simulink model "Labo4_students"  (R2021a)
settings: Solver=VariableStepAuto  StartTime=0.0  StopTime=30.0  RelTol=1e-3
settings Model: Creator=fwielant  LastModifiedBy=sambon
settings SolverCC: AlgebraicLoopSolver=TrustRegion
settings DataIOCC: ReturnWorkspaceOutputs=off
settings DebuggingCC: SFMachineParentedDataDiag=warning  ArithmeticOperatorsInVariantConditions=warning
settings SFSimCC: SimUseLocalCustomCode=off  CustomCodeUndefinedFunction=UseInterfaceOnly
settings RTWCC: RTWUseLocalCustomCode=off  Toolchain=MinGW64 | gmake (64-bit Windows)

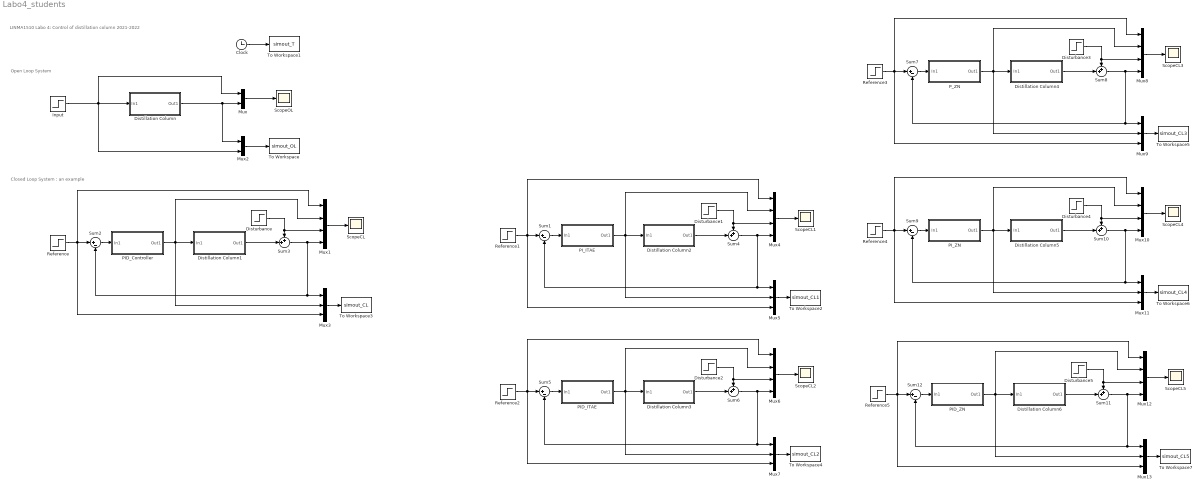
== system Labo4_students ==
  note: Open Loop System
  note: LINMA1510 Labo 4: Control of distillation column 2021-2022
  note: Closed Loop System : an example
  " PID_ITAE" : Subsystem
  Clock : Clock
  Distillation Column : Subsystem
  Distillation Column1 : Subsystem
  Distillation Column2 : Subsystem
  Distillation Column3 : Subsystem
  Distillation Column4 : Subsystem
  Distillation Column5 : Subsystem
  Distillation Column6 : Subsystem
  Disturbance{,1..5} (6 alike) : Step  Time=15  After=0.5  SampleTime=0
  Input : Step  Time=0  SampleTime=0
  Mux : Mux  Inputs=2
  Mux{1,4,6,8,10,12} (6 alike) : Mux
  Mux{3,5,7,9,11,13} (6 alike) : Mux  Inputs=3
  Mux2 : Mux  Inputs=2
  PID_Controller : Subsystem
  PID_ZN : Subsystem
  PI_ITAE : Subsystem
  PI_ZN : Subsystem
  P_ZN : Subsystem
  Reference{,1..5} (6 alike) : Step  SampleTime=0
  ScopeCL{,1..5} (6 alike) : Scope
  ScopeOL : Scope
  Sum{1..2,5,7,9,12} (6 alike) : Sum  Inputs=|+-
  Sum{3..4,6,8,10..11} (6 alike) : Sum  Inputs=++|
  To Workspace : ToWorkspace  VariableName=simout_OL  SampleTime=0.01
      settings: Save2DSignal=2-D array (concatenate along first dimension)
  To Workspace1 : ToWorkspace  VariableName=simout_T  SampleTime=0.01
      settings: Save2DSignal=2-D array (concatenate along first dimension)
  To Workspace2 : ToWorkspace  VariableName=simout_CL1  SampleTime=0.01
      settings: Save2DSignal=2-D array (concatenate along first dimension)
  To Workspace3 : ToWorkspace  VariableName=simout_CL  SampleTime=0.01
      settings: Save2DSignal=2-D array (concatenate along first dimension)
  To Workspace4 : ToWorkspace  VariableName=simout_CL2  SampleTime=0.01
      settings: Save2DSignal=2-D array (concatenate along first dimension)
  To Workspace5 : ToWorkspace  VariableName=simout_CL3  SampleTime=0.01
      settings: Save2DSignal=2-D array (concatenate along first dimension)
  To Workspace6 : ToWorkspace  VariableName=simout_CL4  SampleTime=0.01
      settings: Save2DSignal=2-D array (concatenate along first dimension)
  To Workspace7 : ToWorkspace  VariableName=simout_CL5  SampleTime=0.01
      settings: Save2DSignal=2-D array (concatenate along first dimension)
  wires:
  Input/1 -> Distillation Column/1(In1), Mux2/2, Mux/1
  Mux/1 -> ScopeOL/1
  Sum3/1 -> Sum2/2, Mux3/1, Mux1/4
  Disturbance/1 -> Mux1/3, Sum3/1
  PID_Controller/1(Out1) -> Distillation Column1/1(In1), Mux1/2, Mux3/2
  Reference/1 -> Mux3/3, Mux1/1, Sum2/1
  Sum2/1 -> PID_Controller/1(In1)
  Mux1/1 -> ScopeCL/1
  Mux2/1 -> To Workspace/1
  Mux3/1 -> To Workspace3/1
  Clock/1 -> To Workspace1/1
  Distillation Column/1(Out1) -> Mux/2, Mux2/1
  Distillation Column1/1(Out1) -> Sum3/2
  Disturbance1/1 -> Mux4/3, Sum4/1
  Sum4/1 -> Sum1/2, Mux5/1, Mux4/4
  Mux5/1 -> To Workspace2/1
  Mux4/1 -> ScopeCL1/1
  Reference1/1 -> Mux5/3, Mux4/1, Sum1/1
  Sum1/1 -> PI_ITAE/1(In1)
  PI_ITAE/1(Out1) -> Distillation Column2/1(In1), Mux4/2, Mux5/2
  Distillation Column2/1(Out1) -> Sum4/2
  Disturbance2/1 -> Mux6/3, Sum6/1
  Sum6/1 -> Sum5/2, Mux7/1, Mux6/4
  Mux7/1 -> To Workspace4/1
  Mux6/1 -> ScopeCL2/1
  Reference2/1 -> Mux7/3, Mux6/1, Sum5/1
  Sum5/1 -> " PID_ITAE"/1(In1)
  " PID_ITAE"/1(Out1) -> Distillation Column3/1(In1), Mux6/2, Mux7/2
  Distillation Column3/1(Out1) -> Sum6/2
  Disturbance3/1 -> Mux8/3, Sum8/1
  Sum8/1 -> Sum7/2, Mux9/1, Mux8/4
  Mux9/1 -> To Workspace5/1
  Mux8/1 -> ScopeCL3/1
  Reference3/1 -> Mux9/3, Mux8/1, Sum7/1
  Sum7/1 -> P_ZN/1(In1)
  P_ZN/1(Out1) -> Distillation Column4/1(In1), Mux8/2, Mux9/2
  Distillation Column4/1(Out1) -> Sum8/2
  Distillation Column5/1(Out1) -> Sum10/2
  PI_ZN/1(Out1) -> Distillation Column5/1(In1), Mux10/2, Mux11/2
  Mux10/1 -> ScopeCL4/1
  Reference4/1 -> Mux11/3, Mux10/1, Sum9/1
  Sum9/1 -> PI_ZN/1(In1)
  Disturbance4/1 -> Mux10/3, Sum10/1
  Sum10/1 -> Sum9/2, Mux11/1, Mux10/4
  Mux11/1 -> To Workspace6/1
  Mux13/1 -> To Workspace7/1
  PID_ZN/1(Out1) -> Distillation Column6/1(In1), Mux12/2, Mux13/2
  Reference5/1 -> Mux13/3, Mux12/1, Sum12/1
  Sum11/1 -> Sum12/2, Mux13/1, Mux12/4
  Sum12/1 -> PID_ZN/1(In1)
  Disturbance5/1 -> Mux12/3, Sum11/1
  Mux12/1 -> ScopeCL5/1
  Distillation Column6/1(Out1) -> Sum11/2

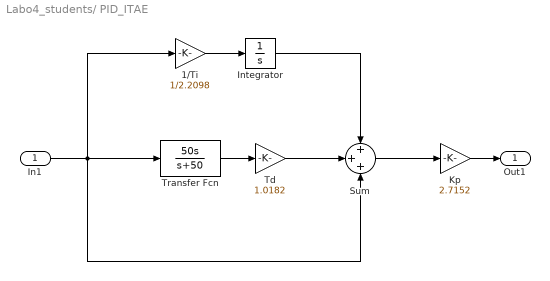
== system Labo4_students/ PID_ITAE ==
  In1 : Inport
  1/Ti : Gain  Gain=1/2.2098
  Integrator : Integrator
  Kp : Gain  Gain=2.7152
  Sum : Sum  Inputs=+++
  Td : Gain  Gain=1.0182
  Transfer Fcn : TransferFcn  Numerator=[50 0]  Denominator=[1 50]
  Out1 : Outport  VectorParamsAs1DForOutWhenUnconnected=off
  wires:
  Sum/1 -> Kp/1
  Kp/1 -> Out1/1
  1/Ti/1 -> Integrator/1
  Integrator/1 -> Sum/1
  In1/1 -> Transfer Fcn/1, Sum/3, 1/Ti/1
  Transfer Fcn/1 -> Td/1
  Td/1 -> Sum/2

== system Labo4_students/Distillation Column ==
  note: ! As Mentionned in the notice of the lab., please avoid to take a look at the model !
  In1 : Inport
  Subsystem : Subsystem
  Out1 : Outport  VectorParamsAs1DForOutWhenUnconnected=off
  wires:
  In1/1 -> Subsystem/1(In1)
  Subsystem/1(Out1) -> Out1/1

== system Labo4_students/Distillation Column1 ==
  note: ! As Mentionned in the notice of the lab., please avoid to take a look at the model !
  In1 : Inport
  Subsystem : Subsystem
  Out1 : Outport  VectorParamsAs1DForOutWhenUnconnected=off
  wires:
  In1/1 -> Subsystem/1(In1)
  Subsystem/1(Out1) -> Out1/1

== system Labo4_students/Distillation Column2 ==
  note: ! As Mentionned in the notice of the lab., please avoid to take a look at the model !
  In1 : Inport
  Subsystem : Subsystem
  Out1 : Outport  VectorParamsAs1DForOutWhenUnconnected=off
  wires:
  In1/1 -> Subsystem/1(In1)
  Subsystem/1(Out1) -> Out1/1

== system Labo4_students/Distillation Column3 ==
  note: ! As Mentionned in the notice of the lab., please avoid to take a look at the model !
  In1 : Inport
  Subsystem : Subsystem
  Out1 : Outport  VectorParamsAs1DForOutWhenUnconnected=off
  wires:
  In1/1 -> Subsystem/1(In1)
  Subsystem/1(Out1) -> Out1/1

== system Labo4_students/Distillation Column4 ==
  note: ! As Mentionned in the notice of the lab., please avoid to take a look at the model !
  In1 : Inport
  Subsystem : Subsystem
  Out1 : Outport  VectorParamsAs1DForOutWhenUnconnected=off
  wires:
  In1/1 -> Subsystem/1(In1)
  Subsystem/1(Out1) -> Out1/1

== system Labo4_students/Distillation Column5 ==
  note: ! As Mentionned in the notice of the lab., please avoid to take a look at the model !
  In1 : Inport
  Subsystem : Subsystem
  Out1 : Outport  VectorParamsAs1DForOutWhenUnconnected=off
  wires:
  In1/1 -> Subsystem/1(In1)
  Subsystem/1(Out1) -> Out1/1

== system Labo4_students/Distillation Column6 ==
  note: ! As Mentionned in the notice of the lab., please avoid to take a look at the model !
  In1 : Inport
  Subsystem : Subsystem
  Out1 : Outport  VectorParamsAs1DForOutWhenUnconnected=off
  wires:
  In1/1 -> Subsystem/1(In1)
  Subsystem/1(Out1) -> Out1/1

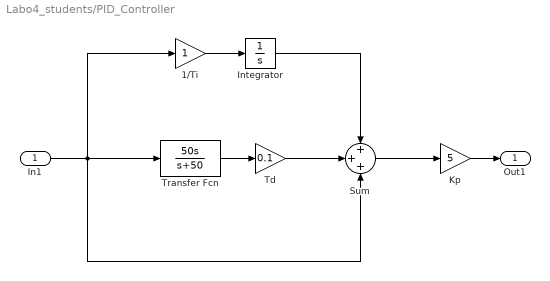
== system Labo4_students/PID_Controller ==
  In1 : Inport
  1/Ti : Gain
  Integrator : Integrator
  Kp : Gain  Gain=5
  Sum : Sum  Inputs=+++
  Td : Gain  Gain=0.1
  Transfer Fcn : TransferFcn  Numerator=[50 0]  Denominator=[1 50]
  Out1 : Outport  VectorParamsAs1DForOutWhenUnconnected=off
  wires:
  Sum/1 -> Kp/1
  Kp/1 -> Out1/1
  1/Ti/1 -> Integrator/1
  Integrator/1 -> Sum/1
  In1/1 -> Transfer Fcn/1, Sum/3, 1/Ti/1
  Transfer Fcn/1 -> Td/1
  Td/1 -> Sum/2

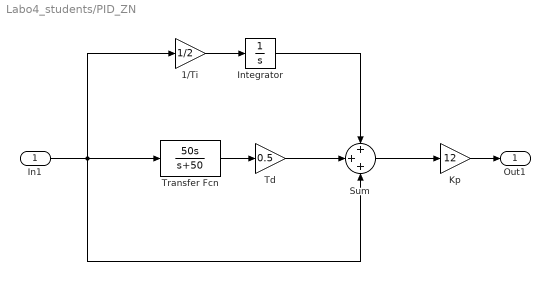
== system Labo4_students/PID_ZN ==
  In1 : Inport
  1/Ti : Gain  Gain=1/2
  Integrator : Integrator
  Kp : Gain  Gain=12
  Sum : Sum  Inputs=+++
  Td : Gain  Gain=0.5
  Transfer Fcn : TransferFcn  Numerator=[50 0]  Denominator=[1 50]
  Out1 : Outport  VectorParamsAs1DForOutWhenUnconnected=off
  wires:
  Sum/1 -> Kp/1
  Kp/1 -> Out1/1
  1/Ti/1 -> Integrator/1
  Integrator/1 -> Sum/1
  In1/1 -> Transfer Fcn/1, Sum/3, 1/Ti/1
  Transfer Fcn/1 -> Td/1
  Td/1 -> Sum/2

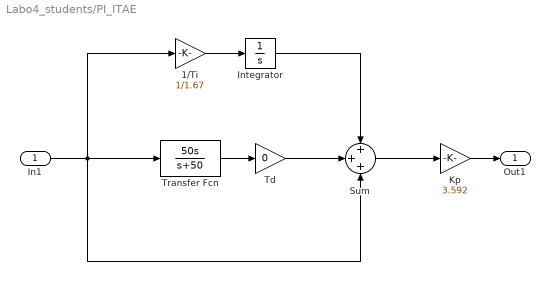
== system Labo4_students/PI_ITAE ==
  In1 : Inport
  1/Ti : Gain  Gain=1/1.67
  Integrator : Integrator
  Kp : Gain  Gain=3.592
  Sum : Sum  Inputs=+++
  Td : Gain  Gain=0
  Transfer Fcn : TransferFcn  Numerator=[50 0]  Denominator=[1 50]
  Out1 : Outport  VectorParamsAs1DForOutWhenUnconnected=off
  wires:
  Sum/1 -> Kp/1
  Kp/1 -> Out1/1
  1/Ti/1 -> Integrator/1
  Integrator/1 -> Sum/1
  In1/1 -> Transfer Fcn/1, Sum/3, 1/Ti/1
  Transfer Fcn/1 -> Td/1
  Td/1 -> Sum/2

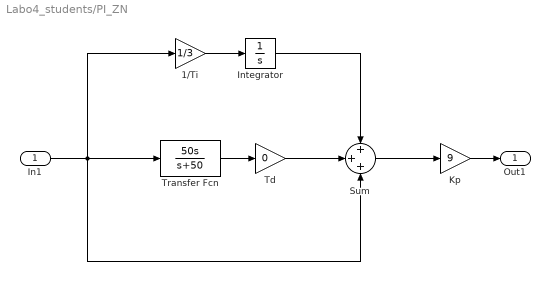
== system Labo4_students/PI_ZN ==
  In1 : Inport
  1/Ti : Gain  Gain=1/3
  Integrator : Integrator
  Kp : Gain  Gain=9
  Sum : Sum  Inputs=+++
  Td : Gain  Gain=0
  Transfer Fcn : TransferFcn  Numerator=[50 0]  Denominator=[1 50]
  Out1 : Outport  VectorParamsAs1DForOutWhenUnconnected=off
  wires:
  Sum/1 -> Kp/1
  Kp/1 -> Out1/1
  1/Ti/1 -> Integrator/1
  Integrator/1 -> Sum/1
  In1/1 -> Transfer Fcn/1, Sum/3, 1/Ti/1
  Transfer Fcn/1 -> Td/1
  Td/1 -> Sum/2

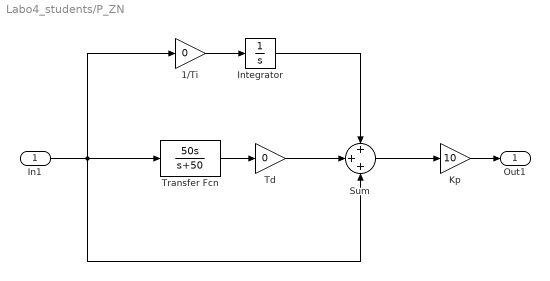
== system Labo4_students/P_ZN ==
  In1 : Inport
  1/Ti : Gain  Gain=0
  Integrator : Integrator
  Kp : Gain  Gain=10
  Sum : Sum  Inputs=+++
  Td : Gain  Gain=0
  Transfer Fcn : TransferFcn  Numerator=[50 0]  Denominator=[1 50]
  Out1 : Outport  VectorParamsAs1DForOutWhenUnconnected=off
  wires:
  Sum/1 -> Kp/1
  Kp/1 -> Out1/1
  1/Ti/1 -> Integrator/1
  Integrator/1 -> Sum/1
  In1/1 -> Transfer Fcn/1, Sum/3, 1/Ti/1
  Transfer Fcn/1 -> Td/1
  Td/1 -> Sum/2

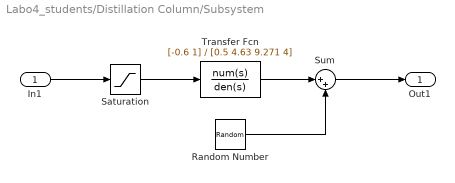
== system Labo4_students/Distillation Column/Subsystem ==
  In1 : Inport
  Random Number : RandomNumber  Variance=0.0001  SampleTime=0.01
  Saturation : Saturate  UpperLimit=15  LowerLimit=-15
  Sum : Sum  Inputs=|++
  Transfer Fcn : TransferFcn  Numerator=[-0.6 1]  Denominator=[0.5 4.63 9.271 4]
  Out1 : Outport  VectorParamsAs1DForOutWhenUnconnected=off
  wires:
  Transfer Fcn/1 -> Sum/1
  Random Number/1 -> Sum/2
  Saturation/1 -> Transfer Fcn/1
  Sum/1 -> Out1/1
  In1/1 -> Saturation/1

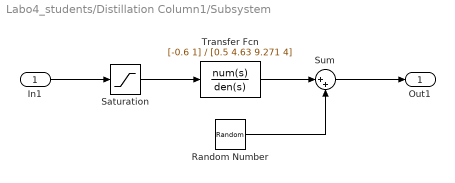
== system Labo4_students/Distillation Column1/Subsystem ==
  In1 : Inport
  Random Number : RandomNumber  Variance=0.0001  SampleTime=0.01
  Saturation : Saturate  UpperLimit=15  LowerLimit=-15
  Sum : Sum  Inputs=|++
  Transfer Fcn : TransferFcn  Numerator=[-0.6 1]  Denominator=[0.5 4.63 9.271 4]
  Out1 : Outport  VectorParamsAs1DForOutWhenUnconnected=off
  wires:
  Transfer Fcn/1 -> Sum/1
  Random Number/1 -> Sum/2
  Saturation/1 -> Transfer Fcn/1
  Sum/1 -> Out1/1
  In1/1 -> Saturation/1

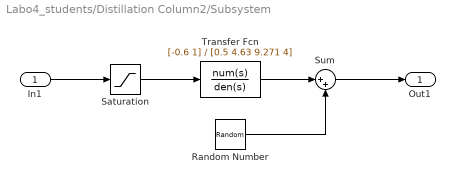
== system Labo4_students/Distillation Column2/Subsystem ==
  In1 : Inport
  Random Number : RandomNumber  Variance=0.0001  SampleTime=0.01
  Saturation : Saturate  UpperLimit=15  LowerLimit=-15
  Sum : Sum  Inputs=|++
  Transfer Fcn : TransferFcn  Numerator=[-0.6 1]  Denominator=[0.5 4.63 9.271 4]
  Out1 : Outport  VectorParamsAs1DForOutWhenUnconnected=off
  wires:
  Transfer Fcn/1 -> Sum/1
  Random Number/1 -> Sum/2
  Saturation/1 -> Transfer Fcn/1
  Sum/1 -> Out1/1
  In1/1 -> Saturation/1

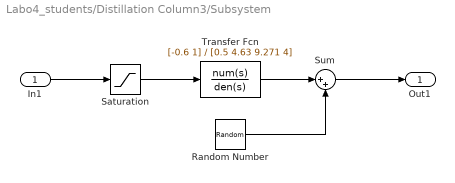
== system Labo4_students/Distillation Column3/Subsystem ==
  In1 : Inport
  Random Number : RandomNumber  Variance=0.0001  SampleTime=0.01
  Saturation : Saturate  UpperLimit=15  LowerLimit=-15
  Sum : Sum  Inputs=|++
  Transfer Fcn : TransferFcn  Numerator=[-0.6 1]  Denominator=[0.5 4.63 9.271 4]
  Out1 : Outport  VectorParamsAs1DForOutWhenUnconnected=off
  wires:
  Transfer Fcn/1 -> Sum/1
  Random Number/1 -> Sum/2
  Saturation/1 -> Transfer Fcn/1
  Sum/1 -> Out1/1
  In1/1 -> Saturation/1

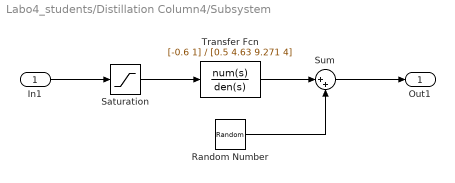
== system Labo4_students/Distillation Column4/Subsystem ==
  In1 : Inport
  Random Number : RandomNumber  Variance=0.0001  SampleTime=0.01
  Saturation : Saturate  UpperLimit=15  LowerLimit=-15
  Sum : Sum  Inputs=|++
  Transfer Fcn : TransferFcn  Numerator=[-0.6 1]  Denominator=[0.5 4.63 9.271 4]
  Out1 : Outport  VectorParamsAs1DForOutWhenUnconnected=off
  wires:
  Transfer Fcn/1 -> Sum/1
  Random Number/1 -> Sum/2
  Saturation/1 -> Transfer Fcn/1
  Sum/1 -> Out1/1
  In1/1 -> Saturation/1

== system Labo4_students/Distillation Column5/Subsystem ==
  In1 : Inport
  Random Number : RandomNumber  Variance=0.0001  SampleTime=0.01
  Saturation : Saturate  UpperLimit=15  LowerLimit=-15
  Sum : Sum  Inputs=|++
  Transfer Fcn : TransferFcn  Numerator=[-0.6 1]  Denominator=[0.5 4.63 9.271 4]
  Out1 : Outport  VectorParamsAs1DForOutWhenUnconnected=off
  wires:
  Transfer Fcn/1 -> Sum/1
  Random Number/1 -> Sum/2
  Saturation/1 -> Transfer Fcn/1
  Sum/1 -> Out1/1
  In1/1 -> Saturation/1

== system Labo4_students/Distillation Column6/Subsystem ==
  In1 : Inport
  Random Number : RandomNumber  Variance=0.0001  SampleTime=0.01
  Saturation : Saturate  UpperLimit=15  LowerLimit=-15
  Sum : Sum  Inputs=|++
  Transfer Fcn : TransferFcn  Numerator=[-0.6 1]  Denominator=[0.5 4.63 9.271 4]
  Out1 : Outport  VectorParamsAs1DForOutWhenUnconnected=off
  wires:
  Transfer Fcn/1 -> Sum/1
  Random Number/1 -> Sum/2
  Saturation/1 -> Transfer Fcn/1
  Sum/1 -> Out1/1
  In1/1 -> Saturation/1
